simulink model "con_ESTHeatingSystem"  (R2017a)
settings: Solver=VariableStepAuto  StartTime=0.0  StopTime=10.0  RelTol=1e-3
settings Model: Creator=xiaodong  LastModifiedBy=xiaodong

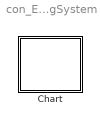
== system con_ESTHeatingSystem ==
  Chart : Stateflow chart  TreatAsAtomicUnit=on

== stateflow chart con_ESTHeatingSystem/Chart ==
  settings: updateMethod=CONTINUOUS
  state M2
    entry:
    A2 = [-0.09961   0.03021   0.03939;
    0.02111   -0.1037    0.0526;
    0.04144   0.05055   -0.1412];
    B2 = [0.03002  -0.001266;
    0.01994     0.8403;
    0.05024  -0.00212];
    during:
  data: u1 function_input; u2 function_input; y function_output; A2 local; B2 local; x local size=3
  data x settings: updateMethod=SF_CONTINUOUS_TIME_DATA
  function y = FnM(u1,u2):
    | function y = FnM(u1,u2)
    | y = u1*u2;
